simulink model "simulink_block_diagram"  (R2021a)
settings: Solver=VariableStepAuto  StartTime=0.0  StopTime=10  MaxStep=1e-4  RelTol=1e-3
undefined symbols (not defined in the file): b1, b2, b3, dx1_0, dx2_0, F_1, F_2, k1, k2, k3, m1, m2, time_F_1, time_F_2, x1_0, x2_0
settings Model: Creator=SPb19  LastModifiedBy=SPb19

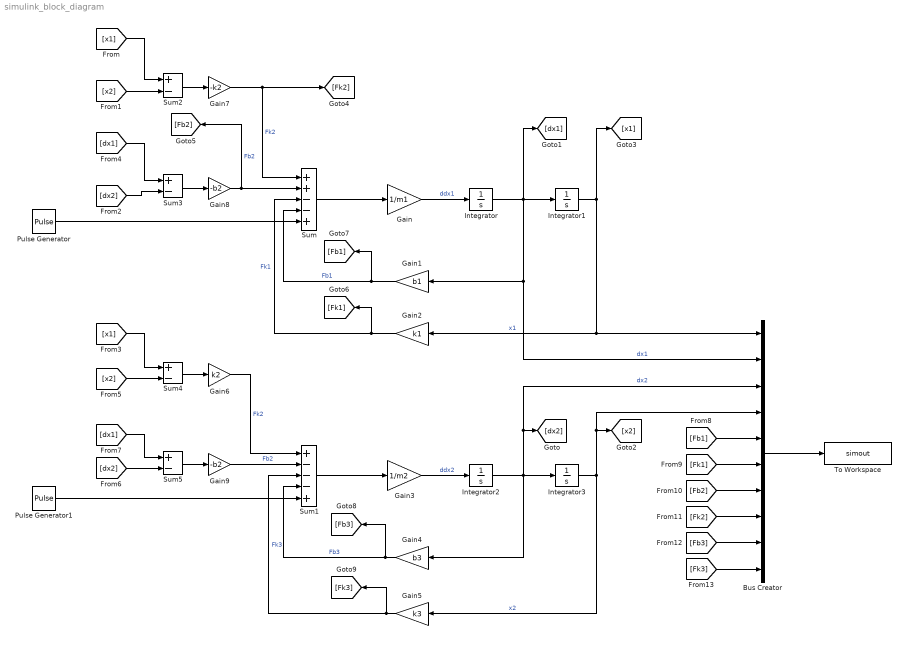
== system simulink_block_diagram ==
  Bus Creator : BusCreator  Inputs=10
  Gain : Gain  Gain=1/m1
  Gain1 : Gain  Gain=b1
  Gain2 : Gain  Gain=k1
  Gain3 : Gain  Gain=1/m2
  Gain4 : Gain  Gain=b3
  Gain5 : Gain  Gain=k3
  Gain6 : Gain  Gain=k2
  Gain7 : Gain  Gain=-k2
  Gain8 : Gain  Gain=-b2
  Gain9 : Gain  Gain=-b2
  Integrator : Integrator  InitialCondition=dx1_0
  Integrator1 : Integrator  InitialCondition=x1_0
  Integrator2 : Integrator  InitialCondition=dx2_0
  Integrator3 : Integrator  InitialCondition=x2_0
  Pulse Generator : DiscretePulseGenerator  PulseType=Time based  Amplitude=F_1  Period=t + 10  PulseWidth=100 * time_F_1 / (t + 10)
  Pulse Generator1 : DiscretePulseGenerator  PulseType=Time based  Amplitude=F_2  Period=t + 10  PulseWidth=100 * time_F_2 / (t + 10)
  Sum : Sum  Inputs=++--+
  Sum1 : Sum  Inputs=+---+
  Sum{2..5} (4 alike) : Sum  Inputs=+-
  To Workspace : ToWorkspace  VariableName=simout  SaveFormat=Timeseries  SampleTime=-1
  wires:
  Integrator1/1 -> Gain2/1, Bus Creator/1, [x1]  "x1"
  Sum/1 -> Gain/1
  Integrator2/1 -> Bus Creator/3, [dx2], Gain4/1, Integrator3/1  "dx2"
  Integrator3/1 -> Bus Creator/4, [x2], Gain5/1  "x2"
  Gain/1 -> Integrator/1  "ddx1"
  Gain3/1 -> Integrator2/1  "ddx2"
  Sum1/1 -> Gain3/1
  Integrator/1 -> [dx1], Bus Creator/2, Gain1/1, Integrator1/1  "dx1"
  Bus Creator/1 -> To Workspace/1
  Gain4/1 -> [Fb3], Sum1/4  "Fb3"
  Gain1/1 -> [Fb1], Sum/4  "Fb1"
  Gain2/1 -> [Fk1], Sum/3  "Fk1"
  Sum2/1 -> Gain7/1
  Gain8/1 -> [Fb2], Sum/2  "Fb2"
  Gain5/1 -> [Fk3], Sum1/3  "Fk3"
  Sum3/1 -> Gain8/1
  Sum4/1 -> Gain6/1
  Sum5/1 -> Gain9/1
  Gain6/1 -> Sum1/1  "Fk2"
  Gain9/1 -> Sum1/2  "Fb2"
  [x2] -> Sum2/2
  [x1] -> Sum2/1
  [dx2] -> Sum3/2
  [dx1] -> Sum3/1
  [x2] -> Sum4/2
  [x1] -> Sum4/1
  [dx2] -> Sum5/2
  [dx1] -> Sum5/1
  Pulse Generator/1 -> Sum/5
  Pulse Generator1/1 -> Sum1/5
  [Fb1] -> Bus Creator/5
  [Fk1] -> Bus Creator/6
  [Fb2] -> Bus Creator/7
  [Fk2] -> Bus Creator/8
  [Fb3] -> Bus Creator/9
  [Fk3] -> Bus Creator/10
  Gain7/1 -> Sum/1, [Fk2]  "Fk2"
